simulink model "Project_O1"  (R2021b)
settings: Solver=VariableStepAuto  StartTime=0.0  StopTime=500  RelTol=1e-3
undefined symbols (not defined in the file): A, B, C1, K, L1
settings Model: Creator=nvnma  LastModifiedBy=nvnma

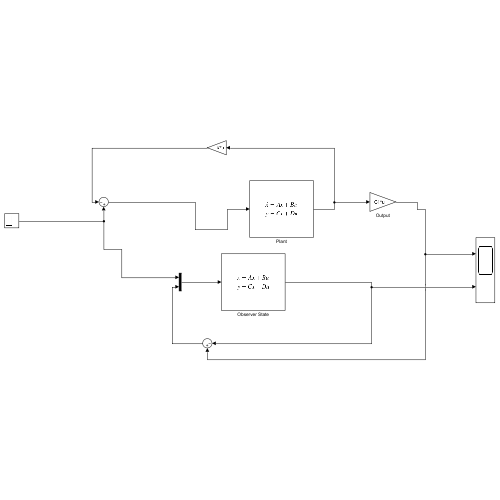
[thumbnail: Simulink's stored preview of the top-level diagram]
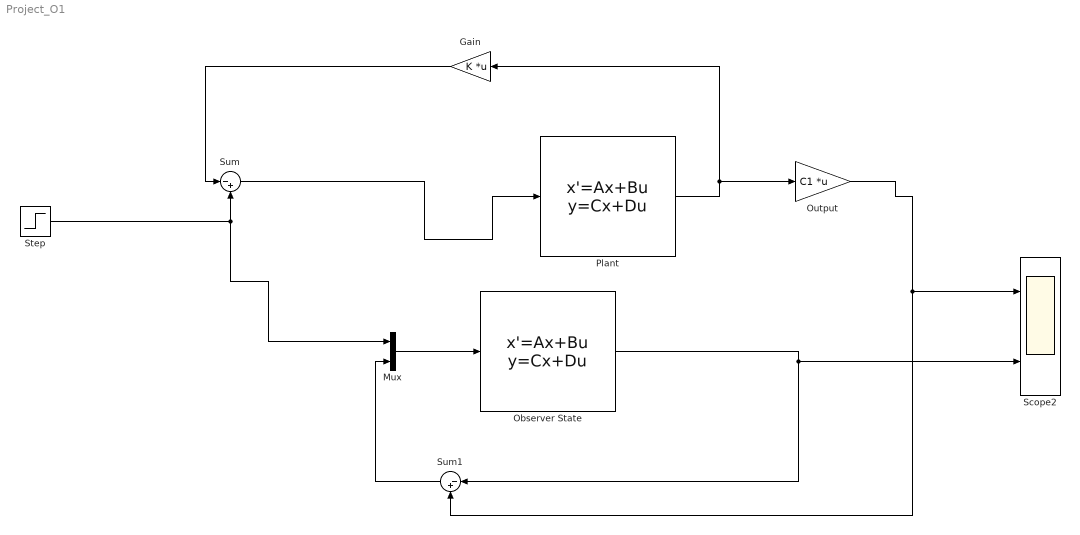
== system Project_O1 ==
  Gain : Gain  Gain=K  Multiplication=Matrix(K*u)
  Mux : Mux  Inputs=2
  Observer State : StateSpace  A=[A - L1*C1]  B=[B L1]  C=C1  D=[0,0]  InitialCondition=[0 0 0 0 0 0]
  Output : Gain  Gain=C1  Multiplication=Matrix(K*u)
  Plant : StateSpace  A=A  B=B  C=eye(6)  D=[0 0 0 0 0 0]'  InitialCondition=[0 0 0 0 0 0]
  Scope2 : Scope  NumInputPorts=2
  Step : Step  SampleTime=0
  Sum : Sum  Inputs=|-+
  Sum1 : Sum  Inputs=|-+
  wires:
  Sum/1 -> Plant/1
  Step/1 -> Mux/1, Sum/2
  Output/1 -> Sum1/2, Scope2/1
  Mux/1 -> Observer State/1
  Plant/1 -> Gain/1, Output/1
  Gain/1 -> Sum/1
  Observer State/1 -> Sum1/1, Scope2/2
  Sum1/1 -> Mux/2
